simulink model "fix_mat_simulink_tb"  (R2021b)
settings: Solver=FixedStepDiscrete  StartTime=0.0  StopTime=1  MaxStep=3.2552083333333335E-6  RelTol=1e-3
model workspace (MAT data in the model file):
  fxpopt_stateflow_dt_s875_g1 : handle (value not decoded)
  fxpopt_stateflow_dt_s876_g2 : handle (value not decoded)
  fxpopt_stateflow_dt_s877_g9 : handle (value not decoded)
  fxpopt_stateflow_dt_s878_g4 : handle (value not decoded)
undefined symbols (not defined in the file or in its folder): img
libraries: dspsrcs4 x1
settings Model: DataTypeOverride=Off  FPTShortcutValueString='{{},{''BaselineRun'',1,1,1,''BaselineRun'','''',{},''M'',''D'',''''},{''EmbeddedRun'',1,1,1,''EmbeddedRun'','''',{},''M'','''',''''},{''BaselineRun_2'',1,1,1,''BaselineRun_2'','''',{},''M'',''D'',''''}}'  Creator=torha  LastModifiedBy=torha
settings OptimizationCC: BlockReduction=off  ConditionallyExecuteInputs=off  DefaultParameterBehavior=Inlined  InheritOutputTypeSmallerThanSingle=on
settings DebuggingCC: SignalRangeChecking=warning  AlgebraicLoopMsg=error  SingleTaskRateTransMsg=error
settings HardwareCC: ProdBitPerPointer=32  ProdBitPerSizeT=32  ProdBitPerPtrDiffT=32  ProdLargestAtomicFloat=None  ProdIntDivRoundTo=Undefined  ProdEndianess=Unspecified  ProdWordSize=32  ProdHWDeviceType=ASIC/FPGA->ASIC/FPGA  TargetBitPerPointer=64  TargetBitPerSizeT=64  TargetBitPerPtrDiffT=64  TargetLongLongMode=on  TargetIntDivRoundTo=Zero  TargetEndianess=LittleEndian  TargetWordSize=64  TargetHWDeviceType=Custom Processor->MATLAB Host Computer  ProdEqTarget=off

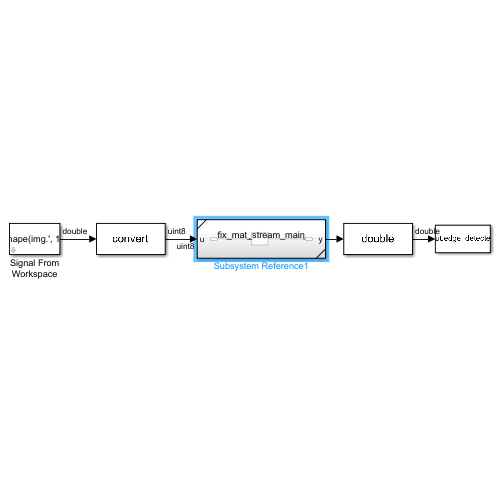
[thumbnail: Simulink's stored preview of the top-level diagram]
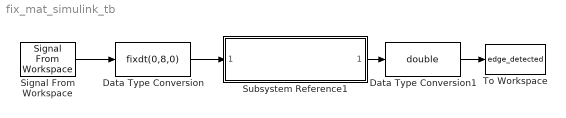
== system fix_mat_simulink_tb ==
  Data Type Conversion : DataTypeConversion  OutMin=0  OutMax=255  OutDataTypeStr=fixdt(0,8,0)
  Data Type Conversion1 : DataTypeConversion  OutDataTypeStr=double
  Signal From Workspace : dspsrcs4/Signal From Workspace  X=reshape(img.', 1, [])  Ts=1/length(img(:))  nsamps=1  OutputAfterFinalValue=Setting to zero  ignoreOrWarnInputAndFrameLengths=off  OutputFrames=off
  Subsystem Reference1 : Subsystem  VariantControl=Choice  ReferencedSubsystem=fix_mat_stream_main
  To Workspace : ToWorkspace  VariableName=edge_detected  SampleTime=-1
  wires:
  Signal From Workspace/1 -> Data Type Conversion/1
  Subsystem Reference1/1 -> Data Type Conversion1/1
  Data Type Conversion/1 -> Subsystem Reference1/1
  Data Type Conversion1/1 -> To Workspace/1
